simulink model "rlmotorDCPIDTune"  (R2021b)
settings: Solver=ode45  StartTime=0.0  StopTime=Inf  RelTol=1e-3  EnableMultiTasking=on
undefined symbols (not defined in the file or in its folder): B, DiscIntNeverNeededParam, J, Ka, Km, L, Q, R, rl, Ts
libraries: rllib x1
settings Model: Creator=The MathWorks, Inc.  LastModifiedBy=ulbio
settings SolverCC: AlgebraicLoopSolver=TrustRegion
settings DataIOCC: LimitDataPoints=on  SaveFormat=Array  SignalLoggingName=logsOut
settings OptimizationCC: ExpressionDepthLimit=2147483647  InitFltsAndDblsToZero=on  LifeSpan=inf
settings DebuggingCC: SaveWithParameterizedLinksMsg=none  UnderspecifiedInitializationDetection=Classic  MergeDetectMultiDrivingBlocksExec=none  SignalResolutionControl=TryResolveAllWithWarning  MultiTaskDSMMsg=warning  FcnCallInpInsideContextMsg=warning  AllowSymbolicDim=off  StateNameClashWarn=warning  SFUnexpectedBacktrackingDiag=warning  SFNoUnconditionalDefaultTransitionDiag=warning  SFExecutionAtInitializationDiag=none  SFMachineParentedDataDiag=warning  ArithmeticOperatorsInVariantConditions=warning
settings HardwareCC: ProdBitPerPointer=32  ProdBitPerSizeT=32  ProdBitPerPtrDiffT=32  ProdLargestAtomicFloat=None  ProdIntDivRoundTo=Undefined  ProdEndianess=Unspecified  ProdWordSize=32  ProdHWDeviceType=Specified
settings ModelReferenceCC: PropagateSignalLabelsOutOfModel=off
settings SFSimCC: SimUseLocalCustomCode=off
settings RTWCC: RTWUseLocalCustomCode=off
settings CodeAppCC: StateflowObjectComments=on
settings GRTTargetCC: TargetFcnLib=ansi_tfl_tmw.mat  TargetLangStandard=C89/C90 (ANSI)  CombineOutputUpdateFcns=off  GRTInterface=on
settings ConfigComp: CovMetricSettings=dw  CovSaveCumulativeToWorkspaceVar=on  CovSaveSingleToWorkspaceVar=on  CovExternalEMLEnable=off

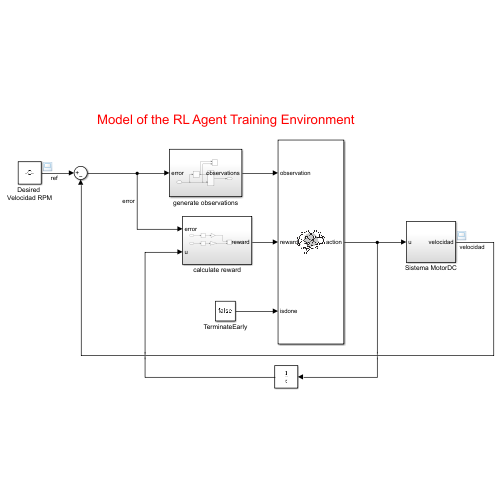
[thumbnail: Simulink's stored preview of the top-level diagram]
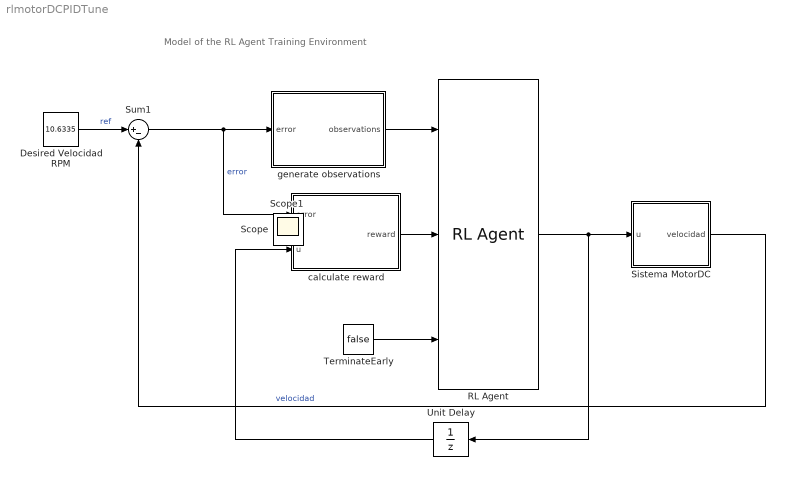
== system rlmotorDCPIDTune ==
  note: Model of the RL Agent Training Environment
  Desired Velocidad RPM : Constant  Value=10.6335
  RL Agent : rllib/RL Agent  Agent=rl.util.PolicyInstance.get('rlmotorDCPIDTune/RL Agent')  ExternalActionAsInput=off  ProvideCumRwd=off  TreatAsDirectFeedthrough=on
  Sistema MotorDC : Subsystem
  Sum1 : Sum  Inputs=|+-  SaturateOnIntegerOverflow=on
  TerminateEarly : Constant  Value=false
  Unit Delay : UnitDelay  SampleTime=-1  HasFrameUpgradeWarning=on
  calculate reward : Subsystem
  generate observations : Subsystem
  Scope : Scope
  Scope1 : Scope
  wires:
  Desired Velocidad RPM/1 -> Sum1/1  "ref"
  Sum1/1 -> calculate reward/1(error), generate observations/1(error)  "error"
  generate observations/1(observations) -> RL Agent/1
  RL Agent/1 -> Unit Delay/1, Sistema MotorDC/1(u)
  Sistema MotorDC/1(velocidad) -> Sum1/2  "velocidad"
  Unit Delay/1 -> calculate reward/2(u)
  calculate reward/1(reward) -> RL Agent/2
  TerminateEarly/1 -> RL Agent/3

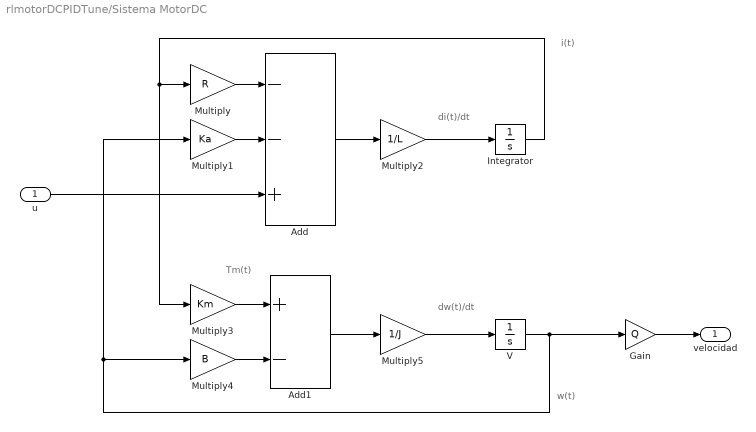
== system rlmotorDCPIDTune/Sistema MotorDC ==
  note: di(t)/dt
  note: w(t)
  note: Tm(t)
  note: i(t)
  note: dw(t)/dt
  u : Inport
  Add : Sum  Inputs=--+
  Add1 : Sum  Inputs=+-
  Gain : Gain  Gain=Q
  Integrator : Integrator
  Multiply : Gain  Gain=R
  Multiply1 : Gain  Gain=Ka
  Multiply2 : Gain  Gain=1/L
  Multiply3 : Gain  Gain=Km
  Multiply4 : Gain  Gain=B
  Multiply5 : Gain  Gain=1/J
  V : Integrator  LimitOutput=on  LowerSaturationLimit=0
  velocidad : Outport  VectorParamsAs1DForOutWhenUnconnected=off
  wires:
  Gain/1 -> velocidad/1
  Integrator/1 -> Multiply3/1, Multiply/1
  Multiply3/1 -> Add1/1
  u/1 -> Add/3
  Multiply2/1 -> Integrator/1
  Multiply1/1 -> Add/2
  Multiply4/1 -> Add1/2
  Add/1 -> Multiply2/1
  Multiply5/1 -> V/1
  V/1 -> Gain/1, Multiply1/1, Multiply4/1
  Multiply/1 -> Add/1
  Add1/1 -> Multiply5/1

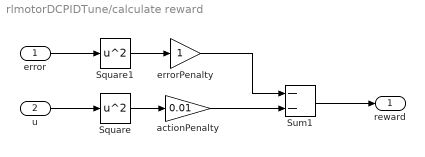
== system rlmotorDCPIDTune/calculate reward ==
  error : Inport
  u : Inport  Port=2
  Square : Math  Operator=square  SaturateOnIntegerOverflow=on
  Square1 : Math  Operator=square  SaturateOnIntegerOverflow=on
  Sum1 : Sum  Inputs=--  OutDataTypeStr=double
  actionPenalty : Gain  Gain=0.01
  errorPenalty : Gain
  reward : Outport  VectorParamsAs1DForOutWhenUnconnected=off
  wires:
  Square1/1 -> errorPenalty/1
  errorPenalty/1 -> Sum1/1
  actionPenalty/1 -> Sum1/2
  Square/1 -> actionPenalty/1
  u/1 -> Square/1
  error/1 -> Square1/1
  Sum1/1 -> reward/1

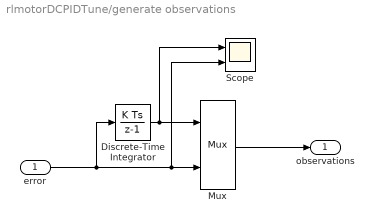
== system rlmotorDCPIDTune/generate observations ==
  error : Inport
  Discrete-Time Integrator : DiscreteIntegrator  SampleTime=Ts  ICPrevOutput=DiscIntNeverNeededParam  ICPrevScaledInput=DiscIntNeverNeededParam
  Mux : Mux  Inputs=2
  Scope : Scope  NumInputPorts=2
  observations : Outport  VectorParamsAs1DForOutWhenUnconnected=off
  wires:
  Discrete-Time Integrator/1 -> Scope/1, Mux/1
  error/1 -> Discrete-Time Integrator/1, Scope/2, Mux/2
  Mux/1 -> observations/1
